simulink model "Problem7_Cascade"  (R2020b)
settings: Solver=VariableStepAuto  StartTime=0.0  StopTime=0.1  RelTol=1e-3
settings Model: Creator=vigne  LastModifiedBy=vigne

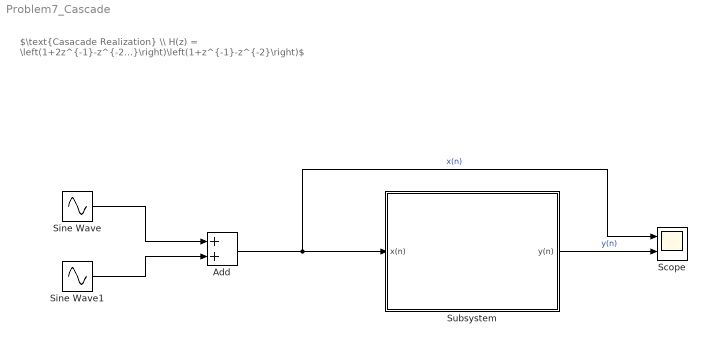
== system Problem7_Cascade ==
  note: $\text{Casacade Realization} \\ H(z) = \left(1+2z^{-1}-z^{-2}\right)\left(1+z^{-1}-z^{-2}\right)$
  Add : Sum
  Scope : Scope  NumInputPorts=2
  Sine Wave : Sin  Frequency=2*pi*30  SampleTime=0
  Sine Wave1 : Sin  Amplitude=0.5  Frequency=2*pi*1000  SampleTime=0
  Subsystem : Subsystem
  wires:
  Add/1 -> Scope/1, Subsystem/1(x(n))  "x(n)"
  Sine Wave/1 -> Add/1
  Subsystem/1(y(n)) -> Scope/2  "y(n)"
  Sine Wave1/1 -> Add/2

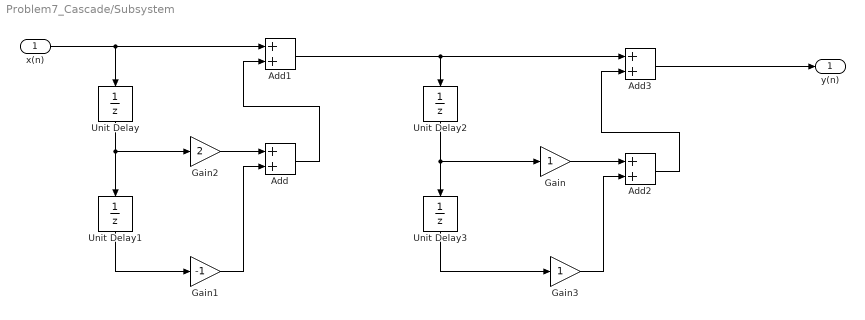
== system Problem7_Cascade/Subsystem ==
  x(n) : Inport
  Add{,1..3} (4 alike) : Sum
  Gain : Gain
  Gain1 : Gain  Gain=-1
  Gain2 : Gain  Gain=2
  Gain3 : Gain
  Unit Delay{,1..3} (4 alike) : UnitDelay  SampleTime=-1  HasFrameUpgradeWarning=on
  y(n) : Outport
  wires:
  Add2/1 -> Add3/2
  Gain2/1 -> Add/1
  Unit Delay/1 -> Unit Delay1/1, Gain2/1
  Unit Delay2/1 -> Gain/1, Unit Delay3/1
  Add/1 -> Add1/2
  Add1/1 -> Unit Delay2/1, Add3/1
  Gain1/1 -> Add/2
  Gain3/1 -> Add2/2
  Gain/1 -> Add2/1
  x(n)/1 -> Add1/1, Unit Delay/1
  Add3/1 -> y(n)/1
  Unit Delay3/1 -> Gain3/1
  Unit Delay1/1 -> Gain1/1
